simulink model "path_tracking"  (R2023b)
settings: Solver=ode4  StartTime=0.0  StopTime=t_end_sim  FixedStep=dt_sim  RelTol=1e-3  EnableMultiTasking=on
values from neighbouring files (symbols this model uses):
  A = A_prec    [main.m]    (also in s_track.m = [(-CF-CR)/(m*Vv),(-CF*a+CR*b-m*Vv^2)/(m*Vv^2))
  a = a_prec    (= 1.3)    [main.m]    (also in s_track.m = a_vet(caso))
  B = B_prec    [main.m]    (also in s_track.m = [CF/(m*Vv) CR/(m*Vv))
  b = b_prec    (= 1.5)    [main.m]    (also in s_track.m = L-a)
  C = eye(4)    [main.m]    (also in s_track.m = [1,0)
  Cf = Cf_prec    (= 120000)    [main.m]
  Cr = Cr_prec    (= 114000)    [main.m]
  D = zeros(4,2)    [main.m]    (also in s_track.m = [0 0)
  disturb_flag = 1    [main.m]
  ff_delay = 0    [main.m]
  G = [   (-Cr-Cf)/(m*V^2),   (-Cf*a+Cr*b)/(m*V^3) ... (first row only)    [main.m]    (also in s_track.m = ss(A,B,C,D))
  H = [Cf/(m*V^2);    1;     Cf/m]    [main.m]
  K_fb = K_feedback_LQR    [main.m]
  K_ff = FeedForward(K_fb)    [main.m]
  K_i = 0    [main.m]
  m = 1575    [main.m]    (also in s_track.m = 2397.12)
  max_delta = max_delta_prec    (= 0.436332312999)    [main.m]
  trajectory_type = 1    [main.m]
  V = V_prec    (= 22.2222222222)    [main.m]    (also in s_track.m = 11.1111111111)
  x0 = 0    [main.m]    (also in s_track.m = X_G(cont1))
settings Model: Creator=gianl  LastModifiedBy=matteo
settings SolverCC: AlgebraicLoopSolver=TrustRegion
settings DataIOCC: ReturnWorkspaceOutputs=off
settings OptimizationCC: LifeSpan=1
settings DebuggingCC: UnconnectedInputMsg=warning  UnconnectedOutputMsg=warning  UnconnectedLineMsg=warning  SFExecutionAtInitializationDiag=none  ArithmeticOperatorsInVariantConditions=warning
settings ModelReferenceCC: EnableRefExpFcnMdlSchedulingChecks=on
settings SFSimCC: SimUseLocalCustomCode=off  CustomCodeUndefinedFunction=UseInterfaceOnly
settings RTWCC: RTWUseLocalCustomCode=off  DLArmComputeVersion=19.05
settings CodeAppCC: StateflowObjectComments=on

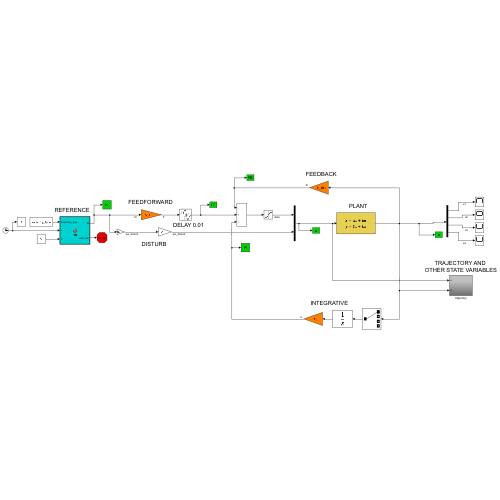
[thumbnail: Simulink's stored preview of the top-level diagram]
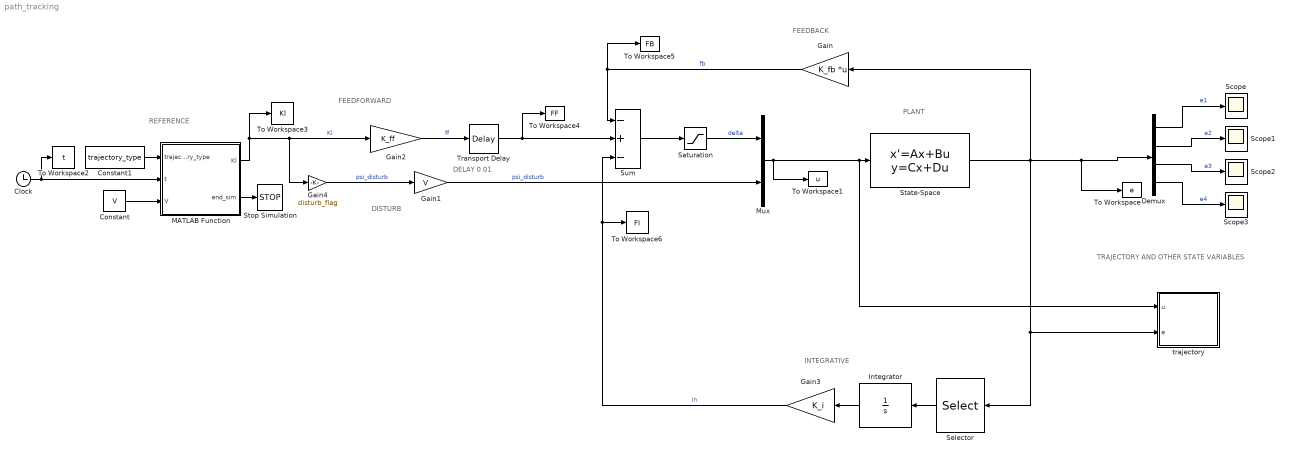
== system path_tracking ==
  note: FEEDBACK
  note: INTEGRATIVE
  note: PLANT
  note: FEEDFORWARD
  note: DISTURB
  note: TRAJECTORY AND
      | OTHER STATE VARIABLES
  note: REFERENCE
  note: DELAY 0.01
  Clock : Clock
  Constant : Constant  Value=V
  Constant1 : Constant  Value=trajectory_type
  Demux : Demux
  Gain : Gain  Gain=K_fb  Multiplication=Matrix(K*u)
  Gain1 : Gain  Gain=V
  Gain2 : Gain  Gain=K_ff
  Gain3 : Gain  Gain=K_i
  Gain4 : Gain  Gain=disturb_flag
  Integrator : Integrator
  MATLAB Function : MATLAB Function  TreatAsAtomicUnit=on
  Mux : Mux  Inputs=2
  Saturation : Saturate  UpperLimit=max_delta  LowerLimit=-max_delta
  Scope{,1..3} (4 alike) : Scope
  Selector : Selector  InputPortWidth=4  IndexOptions=Index vector (dialog)  Indices=[1]  OutputSizes=1
  State-Space : StateSpace  A=A  B=B  C=C  D=D  InitialCondition=x0  ParameterTunability=Unconstrained
  Stop Simulation : Stop
  Sum : Sum  Inputs=-+-
  To Workspace : ToWorkspace  VariableName=e  SampleTime=-1
  To Workspace1 : ToWorkspace  VariableName=u  SampleTime=-1
  To Workspace2 : ToWorkspace  VariableName=t  SampleTime=-1
  To Workspace3 : ToWorkspace  VariableName=Kl  SampleTime=-1
  To Workspace4 : ToWorkspace  VariableName=FF  SampleTime=-1
  To Workspace5 : ToWorkspace  VariableName=FB  SampleTime=-1
  To Workspace6 : ToWorkspace  VariableName=FI  SampleTime=-1
  Transport Delay : TransportDelay  DelayTime=ff_delay
  trajectory : Subsystem
  wires:
  Demux/1 -> Scope/1  "e1"
  Demux/2 -> Scope1/1  "e2"
  Demux/3 -> Scope2/1  "e3"
  Demux/4 -> Scope3/1  "e4"
  Gain1/1 -> Mux/2  "psi_disturb"
  Clock/1 -> To Workspace2/1, MATLAB Function/2(t)
  Gain/1 -> To Workspace5/1, Sum/1  "fb"
  Sum/1 -> Saturation/1
  MATLAB Function/1(Kl) -> Gain2/1, Gain4/1, To Workspace3/1  "Kl"
  Gain2/1 -> Transport Delay/1  "ff"
  Saturation/1 -> Mux/1  "delta"
  Constant1/1 -> MATLAB Function/1(trajectory_type)
  Constant/1 -> MATLAB Function/3(V)
  MATLAB Function/2(end_sim) -> Stop Simulation/1
  Selector/1 -> Integrator/1
  Integrator/1 -> Gain3/1
  Gain3/1 -> To Workspace6/1, Sum/3  "in"
  Mux/1 -> To Workspace1/1, trajectory/1(u), State-Space/1
  State-Space/1 -> trajectory/2(e), Selector/1, Gain/1, Demux/1, To Workspace/1
  Transport Delay/1 -> Sum/2, To Workspace4/1
  Gain4/1 -> Gain1/1  "psi_disturb"

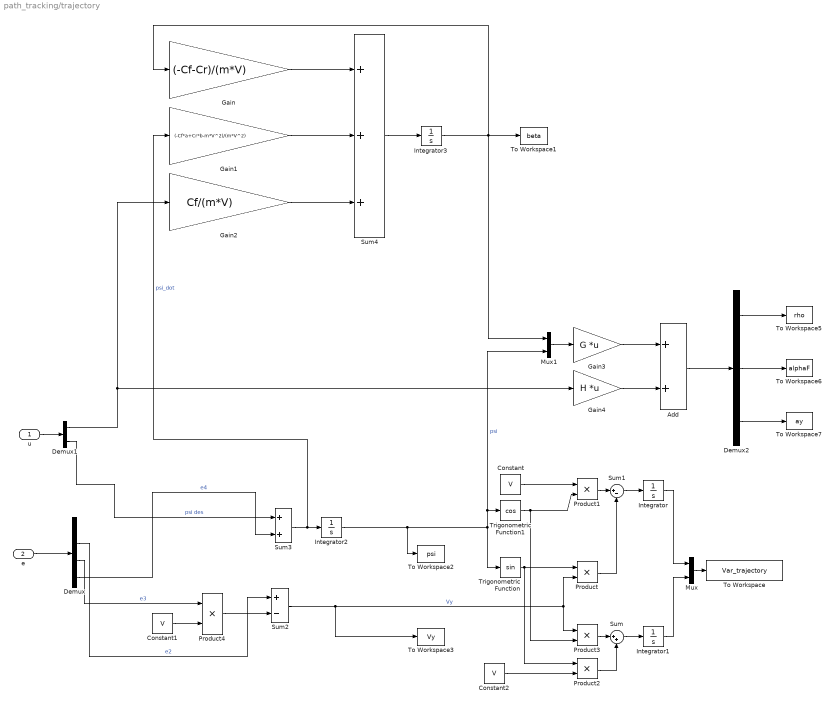
== system path_tracking/trajectory ==
  u : Inport
  e : Inport  Port=2
  Add : Sum
  Constant : Constant  Value=V
  Constant1 : Constant  Value=V
  Constant2 : Constant  Value=V
  Demux : Demux
  Demux1 : Demux  Outputs=2
  Demux2 : Demux  Outputs=3
  Gain : Gain  Gain=(-Cf-Cr)/(m*V)
  Gain1 : Gain  Gain=(-Cf*a+Cr*b-m*V^2)/(m*V^2)
  Gain2 : Gain  Gain=Cf/(m*V)
  Gain3 : Gain  Gain=G  Multiplication=Matrix(K*u)
  Gain4 : Gain  Gain=H  Multiplication=Matrix(K*u)
  Integrator{,1..3} (4 alike) : Integrator
  Mux : Mux  Inputs=2
  Mux1 : Mux  Inputs=2
  Product{,1..3} (4 alike) : Product  InputSameDT=on  SaturateOnIntegerOverflow=on  OutDataTypeStr=Inherit: Same as first input
  Product4 : Product
  Sum : Sum  Inputs=|++  InputSameDT=on  SaturateOnIntegerOverflow=on  OutDataTypeStr=Inherit: Same as first input
  Sum1 : Sum  Inputs=|+-  InputSameDT=on  SaturateOnIntegerOverflow=on  OutDataTypeStr=Inherit: Same as first input
  Sum2 : Sum  Inputs=+-
  Sum3 : Sum
  Sum4 : Sum  Inputs=+++
  To Workspace : ToWorkspace  VariableName=Var_trajectory  SampleTime=-1
      settings: Save2DSignal=2-D array (concatenate along first dimension)
      settings: InitFcn=|
      | ParentName = get_param(gcb,'Parent');
      | cont = max(find(ParentName=='/'));
      | set_param(gcb,'VariableName',strcat('Var_',ParentName(cont+1:length(ParentName))));
      | clear ParentName cont
  To Workspace1 : ToWorkspace  VariableName=beta  SampleTime=-1
  To Workspace2 : ToWorkspace  VariableName=psi  SampleTime=-1
  To Workspace3 : ToWorkspace  VariableName=Vy  SampleTime=-1
  To Workspace5 : ToWorkspace  VariableName=rho  SampleTime=-1
  To Workspace6 : ToWorkspace  VariableName=alphaF  SampleTime=-1
  To Workspace7 : ToWorkspace  VariableName=ay  SampleTime=-1
  Trigonometric Function : Trigonometry
  Trigonometric Function1 : Trigonometry  Operator=cos
  wires:
  Product1/1 -> Sum1/1
  Product/1 -> Sum1/2
  Sum1/1 -> Integrator/1
  Trigonometric Function/1 -> Product/1, Product2/1
  Constant/1 -> Product1/1
  Sum2/1 -> Product/2, Product3/1, To Workspace3/1  "Vy"
  Trigonometric Function1/1 -> Product1/2, Product3/2
  Product3/1 -> Sum/1
  Product2/1 -> Sum/2
  Sum/1 -> Integrator1/1
  Integrator/1 -> Mux/1
  Integrator1/1 -> Mux/2
  Mux/1 -> To Workspace/1
  Integrator2/1 -> To Workspace2/1, Mux1/2, Trigonometric Function1/1, Trigonometric Function/1  "psi"
  Constant1/1 -> Product4/2
  Product4/1 -> Sum2/2
  Demux1/2 -> Sum3/1  "psi des"
  Sum3/1 -> Gain1/1, Integrator2/1  "psi_dot"
  e/1 -> Demux/1
  Constant2/1 -> Product2/2
  Demux/2 -> Sum2/1  "e2"
  Demux/3 -> Product4/1  "e3"
  Demux/4 -> Sum3/2  "e4"
  Integrator3/1 -> Gain/1, To Workspace1/1, Mux1/1
  Sum4/1 -> Integrator3/1
  Gain/1 -> Sum4/1
  Gain1/1 -> Sum4/2
  Gain2/1 -> Sum4/3
  u/1 -> Demux1/1
  Demux1/1 -> Gain2/1, Gain4/1
  Mux1/1 -> Gain3/1
  Gain3/1 -> Add/1
  Gain4/1 -> Add/2
  Add/1 -> Demux2/1
  Demux2/1 -> To Workspace5/1
  Demux2/2 -> To Workspace6/1
  Demux2/3 -> To Workspace7/1

== matlab function path_tracking/MATLAB Function ==
  data: trajectory_type input; t input; Kl output; V input; end_sim output
function [Kl, end_sim] = fcn(trajectory_type, t, V)

Kl = 0;
end_sim = 0;

max_kl = 2e-3;
if trajectory_type == 1  % EXAMPLE
    t1=10;
    t2=20;
    t3=40;
    t4=50;
    t5=60;
    t6=70;
    t7=90;
    t8=100;
    
    if t<t1 
        Kl = 0;
    elseif t < t2
        Kl = -max_kl/(t2-t1) *(t-t1);
    elseif t < t3
        Kl = -max_kl;
    elseif t < t4
        Kl = -max_kl + max_kl/(t4-t3) *(t-t3);
    elseif t < t5
        Kl = 0;
    elseif t < t6
        Kl = max_kl/(t6-t5) *(t-t5);
    elseif t < t7
        Kl = max_kl;
    elseif t < t8
        Kl = max_kl - max_kl/(t8-t7) *(t-t7);
    elseif t > t8+2
        end_sim = 1;
    end
end
%% CIRCLE
if trajectory_type == 2
    R = 500;
    Kl = 1/R;
    if t > 2*pi*R/V 
        end_sim = 1;
    end
end
%% LOOP
if trajectory_type == 3 
    R = 500;
    t_semicirc = pi*R/V;
    if t < t_semicirc || t > 3 *t_semicirc
        Kl = 1/R; 
    else
        Kl = -1/R;
    end

    if t > 4*t_semicirc
        end_sim = 1;
    end
end
%% SORPASSO
if trajectory_type == 4
    max_kl = max_kl/100;
    t1=10;
    t2=t1+2;
    t3=t2+10;
    t4=t3+2;
    t5=t4+10;
    t6=t5+2;
    t7=t6+10;
    t8=t7+2;

    t10=t8+20;
    t20=t10+2;
    t30=t20+10;
    t40=t30+2;
    t50=t40+10;
    t60=t50+2;
    t70=t60+10;
    t80=t70+2;
    
    if t<t1
        Kl = 0;
    elseif t < t2
        Kl = -max_kl/(t2-t1) *(t-t1);
    elseif t < t3
        Kl = -max_kl;
    elseif t < t4
        Kl = -max_kl + max_kl/(t4-t3) *(t-t3);
    elseif t < t5
        Kl = 0;
    elseif t < t6
        Kl = max_kl/(t6-t5) *(t-t5);
    elseif t < t7
        Kl = max_kl;
    elseif t < t8
        Kl = max_kl - max_kl/(t8-t7) *(t-t7);
    elseif t<t10
        Kl = 0;
    elseif t < t20
        Kl = +max_kl/(t20-t10) *(t-t10);
    elseif t < t30
        Kl = max_kl;
    elseif t < t40
        Kl = max_kl - max_kl/(t40-t30) *(t-t30);
    elseif t < t50
        Kl = 0;
    elseif t < t60
        Kl = -max_kl/(t60-t50) *(t-t50);
    elseif t < t70
        Kl = -max_kl;
    elseif t < t80
        Kl = -max_kl + max_kl/(t80-t70) *(t-t70);
    end

    if t > t80+2
        end_sim = 1;
    end
end
%% STEP INPUT 
if trajectory_type == 5
    if t<10
        Kl = 0;
    else
        Kl = 1;
    end
    if t > 50
        end_sim = 1;
    end
end
